simulink model "simulink_example_loil"  (R2020b)
settings: Solver=VariableStepAuto  StartTime=0.0  StopTime=10.0  RelTol=1e-3
undefined symbols (not defined in the file): c, k, k2, m, x0
settings Model: Creator=rrb32  LastModifiedBy=rrb32

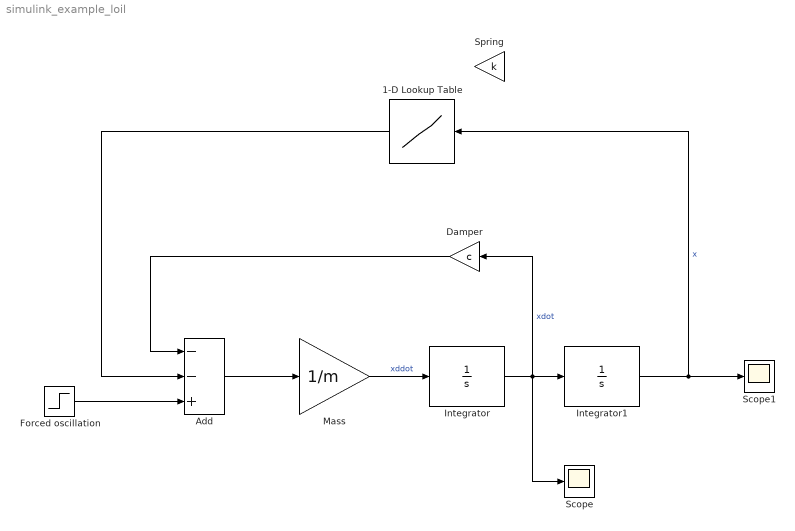
== system simulink_example_loil ==
  1-D Lookup Table : Lookup_n-D  NumberOfTableDimensions=1  BreakpointsForDimension1=[(-2*x0), -x0, x0, (2*x0)]  Table=[-(k+k2)*x0,-k*x0,k*x0,(k+k2)*x0]  InternalRulePriority=Speed  RndMeth=Simplest  InputSameDT=on
  Add : Sum  Inputs=--+
  Damper : Gain  Gain=c
  Forced oscillation : Step  After=1000  SampleTime=0
  Integrator : Integrator
  Integrator1 : Integrator
  Mass : Gain  Gain=1/m
  Scope : Scope
  Scope1 : Scope
  Spring : Gain  Gain=k
  wires:
  Integrator/1 -> Scope/1, Damper/1, Integrator1/1  "xdot"
  Mass/1 -> Integrator/1  "xddot"
  Integrator1/1 -> 1-D Lookup Table/1, Scope1/1  "x"
  Damper/1 -> Add/1
  Add/1 -> Mass/1
  Forced oscillation/1 -> Add/3
  1-D Lookup Table/1 -> Add/2
